simulink model "ZT_VehCtrl_18B"  (R2018b)
settings: Solver=FixedStepAuto  StartTime=0.0  StopTime=inf  FixedStep=0.005  RelTol=1e-3
InitFcn:
  | mbd_mpc_consistency_checks(bdroot(gcs));
undefined symbols (not defined in the file or in its folder): ANG_DEAD, BMS_NormalPwr, BrkPrsByBrkPct_TB_X, BrkPrsByBrkPct_TB_Y, DELAY_DISCHARGE, DELAY_RCUOFF, DRV_BACKWARD, DRV_BRAKE, DRV_FORWARD, DRV_NEUTRAL, DRV_PARK, DRV_UNPARK, DRV_ZEROTURN, EPB_LOCK, EPB_UNLOCK, ExtraLoadPwr, FanOff, fifo_0_vect, fifo_1_vect, HiFanReq, HV_finished, HV_No_Active, HV_POWER_OFF, HV_POWER_ON, HVDown, HVON, KaTLS_v_DrgUp_X_VehSpd, KeFTM_s_Way1OffDlyTime, KeFTM_TK_Way1CoolLv2OffBatTemp, KeFTM_TK_Way1CoolLv2OffMtrTemp, KeFTM_TK_Way1CoolLv2OnBatTemp, KeFTM_TK_Way1CoolLv2OnMtrTemp, KeFTM_TK_Way1CoolLv3OffBatTemp, KeFTM_TK_Way1CoolLv3OffMtrTemp, KeFTM_TK_Way1CoolLv3OnBatTemp, KeFTM_TK_Way1CoolLv3OnMtrTemp, KeFTM_TK_Way1CoolLv4OffBatTemp, KeFTM_TK_Way1CoolLv4OffMtrTemp, KeFTM_TK_Way1CoolLv4OnBatTemp, KeFTM_TK_Way1CoolLv4OnMtrTemp, Kp1, Kp2, LowFanReq, LQFP, MtrPwrFactor_RCU, MtrPwrHighToMidThd, MtrPwrLowToMidThd, MtrPwrMidToHighThd, MtrPwrMidToLowThd, MtrTrqMax, PCT_DEAD, Precharge, PTO_1000, PTO_540, pts1_fifo_0_vect, pts1_fifo_1_vect, pts2_fifo_0_vect, pts2_fifo_1_vect, pts3_fifo_0_vect, pts3_fifo_1_vect ... (+24)
libraries: mbd_mpc574x_ec_toolbox x173, canmsglib x72, simulink x57
(part 10 of 12)

== system ZT_VehCtrl_18B/SigIn/CAN1/TWV /UNPACK ==
  ID : Inport
  data : Inport  Port=2
  length : Inport  Port=3
  timestamp : Inport  Port=4
  Action Port : ActionPort
  Bus Creator : BusCreator  Inputs=7  OutDataTypeStr=Bus: CAN_MESSAGE_BUS  NonVirtualBus=on
  Bus Creator1 : BusCreator  Inputs=3
  CAN Unpack6 : canmsglib/CAN Unpack  CANdbFile=D:\VCU\VCU_SL_ZhengZhou\ZT2\模型与接口\CAN_DBC\动力CANB_GBK.dbc  MsgList=TWV  MsgName=TWV  MsgIDType=Extended (29-bit identifier)  MsgIdentifier=419374139  MsgLength=8  SignalInfo=TWV1_P_MotorOpenCircuitFlt$6$1$1$2$1$0$1$0$0$1$#TWV1_P_MotorSta$7$1$1$2$1$0$1$0$0$1$#TWV1_P_OverCurrent$2$1$1$2$1$0$1$0$0$1$#TWV1_P_OverTempFlt$3$1$1$2$1$0$1$0$0$1$#TWV1_P_OverVoltageFlt$1$1$1$2$1$0$1$0$0$1$#TWV1_P_RESP_ERROR$0$1$1$2$1$0$1$0$0$1$#TWV1_P_RealSta$8$8$1$2$1$0$4.000000e-01$0$0$100$#TWV1_P_StallFlt$5$1$1$2$1$0$1$0$0$1$#TWV1_P_UnderVoltageFlt$4$1$1$2$1$0$1$0$0$1$#  NSignals=9  IDPort=off  TimestampPort=off  ErrorPort=off  RemotePort=off  LengthPort=off  StatusPort=off  StartBits=str2num('[int32(6);int32(7);int32(2);int32(3);int32(1);int32(0);int32(8);int32(5);int32(4)]')  SignalSizes=str2num('[int32(1);int32(1);int32(1);int32(1);int32(1);int32(1);int32(8);int32(1);int32(1)]')  ByteOrders=str2num('[int32(1);int32(1);int32(1);int32(1);int32(1);int32(1);int32(1);int32(1);int32(1)]')  DataTypes=str2num('[int32(2);int32(2);int32(2);int32(2);int32(2);int32(2);int32(2);int32(2);int32(2)]')  MultiplexTypes=str2num('[int32(1);int32(1);int32(1);int32(1);int32(1);int32(1);int32(1);int32(1);int32(1)]')  MultiplexValues=str2num('[double(0);double(0);double(0);double(0);double(0);double(0);double(0);double(0);double(0)]')  Factors=str2num('[double(1);double(1);double(1);double(1);double(1);double(1);double(4.000000e-01);double(1);double(1)]')  Offsets=str2num('[double(0);double(0);double(0);double(0);double(0);double(0);double(0);double(0);double(0)]')  Minimums=str2num('[double(0);double(0);double(0);double(0);double(0);double(0);double(0);double(0);double(0)]')  Maximums=str2num('[double(1);double(1);double(1);double(1);double(1);double(1);double(100);double(1);double(1)]')  ApplyMinMax=off
      settings: SourceProductName=Simulink Real-Time  SourceProductBaseCode=XP  DataFormat=CANdb specified signals
  Constant1 : Constant  OutDataTypeStr=uint8
  Constant4 : Constant  Value=0  OutDataTypeStr=uint8
  Constant5 : Constant  Value=0  OutDataTypeStr=uint8
  Data Type Conversion{,14..15,17} (4 alike) : DataTypeConversion  OutDataTypeStr=uint8
  Data Type Conversion18 : DataTypeConversion  OutDataTypeStr=uint32
  Data Type Conversion19 : DataTypeConversion  OutDataTypeStr=double
  Message : Outport
  wires:
  Constant4/1 -> Data Type Conversion15/1
  length/1 -> Data Type Conversion14/1
  data/1 -> Bus Creator/7  "Data"
  Data Type Conversion18/1 -> Bus Creator/5  "ID"
  Constant1/1 -> Data Type Conversion/1
  Constant5/1 -> Data Type Conversion17/1
  ID/1 -> Data Type Conversion18/1
  Data Type Conversion19/1 -> Bus Creator/6  "Timestamp"
  timestamp/1 -> Data Type Conversion19/1
  Data Type Conversion17/1 -> Bus Creator/4  "Error"
  Bus Creator/1 -> CAN Unpack6/1  "CAN_Msg_In"
  Data Type Conversion/1 -> Bus Creator/1  "Extended"
  Data Type Conversion14/1 -> Bus Creator/2  "Length"
  Data Type Conversion15/1 -> Bus Creator/3  "Remote"
  Bus Creator1/1 -> Message/1

== system ZT_VehCtrl_18B/SigIn/PWM/PWM_PTS1/Subsystem ==
  In1 : Inport
  Add2 : Sum  AccumDataTypeStr=single
  Constant : Constant  OutDataTypeStr=uint8
  Constant1 : Constant  Value=0  OutDataTypeStr=single
  Data Store Read3 : DataStoreRead  DataStoreName=pts1_pwm_cnt
  Data Store Write : DataStoreWrite  DataStoreName=pts1_pwm_cnt
  Saturation : Saturate  UpperLimit=100  LowerLimit=0
  Switch : Switch  Criteria=u2 > Threshold  Threshold=100
  Out1 : Outport  VectorParamsAs1DForOutWhenUnconnected=on
  wires:
  Saturation/1 -> Data Store Write/1
  Add2/1 -> Switch/2, Saturation/1
  Data Store Read3/1 -> Add2/2
  Constant1/1 -> Switch/1
  Switch/1 -> Out1/1
  Constant/1 -> Add2/1
  In1/1 -> Switch/3

== system ZT_VehCtrl_18B/SigIn/PWM/PWM_PTS1/Subsystem_capture ==
  In1 : Inport
  function : TriggerPort  TriggerType=function-call  VariantControl=Variant
  Constant : Constant  Value=0  OutDataTypeStr=uint8
  Counter Limited : simulink/Sources/Counter Limited  uplimit=7  tsamp=-1
  Data Store Write : DataStoreWrite  DataStoreName=pts1_pwm_cnt
  Data Store Write3 : DataStoreWrite  DataStoreName=pwm3_cnt
  Terminator : Terminator
  eTimer_Arm_Capture : mbd_mpc574x_ec_toolbox/Motor Control Blocks/eTIMER Blocks/eTimer_Arm_Capture  etimerModule=1  etimerChannel=2  etimerArmAction=Stop
  eTimer_Capture : mbd_mpc574x_ec_toolbox/Motor Control Blocks/eTIMER Blocks/eTimer_Capture  etimerModule=1  etimerChannel=2
      settings: SourceProductName=NXP Model-Based Design Toolbox for MPC57xx MCUs
  Out1 : Outport  OutDataTypeStr=uint16
  Out2 : Outport  Port=2  OutDataTypeStr=uint16
  Out3 : Outport  Port=3  OutDataTypeStr=uint16
  Out4 : Outport  Port=4  OutDataTypeStr=uint16
  wires:
  eTimer_Capture/1 -> Out1/1
  eTimer_Capture/4 -> Out4/1
  eTimer_Capture/3 -> Out3/1
  eTimer_Capture/2 -> Out2/1
  In1/1 -> Terminator/1
  Constant/1 -> Data Store Write/1
  Counter Limited/1 -> Data Store Write3/1

== system ZT_VehCtrl_18B/SigIn/PWM/PWM_PTS2/Subsystem ==
  In1 : Inport
  Add2 : Sum  AccumDataTypeStr=single
  Constant : Constant  OutDataTypeStr=uint8
  Constant1 : Constant  Value=0  OutDataTypeStr=single
  Data Store Read3 : DataStoreRead  DataStoreName=pts2_pwm_cnt
  Data Store Write : DataStoreWrite  DataStoreName=pts2_pwm_cnt
  Saturation : Saturate  UpperLimit=100  LowerLimit=0
  Switch : Switch  Criteria=u2 > Threshold  Threshold=100
  Out1 : Outport  VectorParamsAs1DForOutWhenUnconnected=on
  wires:
  In1/1 -> Switch/3
  Constant/1 -> Add2/1
  Switch/1 -> Out1/1
  Constant1/1 -> Switch/1
  Data Store Read3/1 -> Add2/2
  Add2/1 -> Saturation/1, Switch/2
  Saturation/1 -> Data Store Write/1

== system ZT_VehCtrl_18B/SigIn/PWM/PWM_PTS2/Subsystem_capture ==
  In1 : Inport
  function : TriggerPort  TriggerType=function-call  VariantControl=Variant
  Constant : Constant  Value=0  OutDataTypeStr=uint8
  Counter Limited : simulink/Sources/Counter Limited  uplimit=255  tsamp=-1
  Data Store Write : DataStoreWrite  DataStoreName=pts2_pwm_cnt
  Data Store Write2 : DataStoreWrite  DataStoreName=pwm2_cnt
  Terminator : Terminator
  eTimer_Arm_Capture : mbd_mpc574x_ec_toolbox/Motor Control Blocks/eTIMER Blocks/eTimer_Arm_Capture  etimerModule=1  etimerChannel=3  etimerArmAction=Stop
  eTimer_Capture : mbd_mpc574x_ec_toolbox/Motor Control Blocks/eTIMER Blocks/eTimer_Capture  etimerModule=1  etimerChannel=3
      settings: SourceProductName=NXP Model-Based Design Toolbox for MPC57xx MCUs
  Out1 : Outport  OutDataTypeStr=uint16
  Out2 : Outport  Port=2  OutDataTypeStr=uint16
  Out3 : Outport  Port=3  OutDataTypeStr=uint16
  Out4 : Outport  Port=4  OutDataTypeStr=uint16
  wires:
  Constant/1 -> Data Store Write/1
  In1/1 -> Terminator/1
  eTimer_Capture/2 -> Out2/1
  eTimer_Capture/3 -> Out3/1
  eTimer_Capture/4 -> Out4/1
  eTimer_Capture/1 -> Out1/1
  Counter Limited/1 -> Data Store Write2/1

== system ZT_VehCtrl_18B/SigIn/PWM/PWM_PTS3/Subsystem ==
  In1 : Inport
  Add2 : Sum  AccumDataTypeStr=single
  Constant : Constant  OutDataTypeStr=uint8
  Constant1 : Constant  Value=0  OutDataTypeStr=single
  Data Store Read3 : DataStoreRead  DataStoreName=pts3_pwm_cnt
  Data Store Write : DataStoreWrite  DataStoreName=pts3_pwm_cnt
  Saturation : Saturate  UpperLimit=100  LowerLimit=0
  Switch : Switch  Criteria=u2 > Threshold  Threshold=100
  Out1 : Outport  VectorParamsAs1DForOutWhenUnconnected=on
  wires:
  Saturation/1 -> Data Store Write/1
  Add2/1 -> Switch/2, Saturation/1
  Data Store Read3/1 -> Add2/2
  Constant1/1 -> Switch/1
  Switch/1 -> Out1/1
  Constant/1 -> Add2/1
  In1/1 -> Switch/3

== system ZT_VehCtrl_18B/SigIn/PWM/PWM_PTS3/Subsystem_capture ==
  In1 : Inport
  function : TriggerPort  TriggerType=function-call  VariantControl=Variant
  Constant : Constant  Value=0  OutDataTypeStr=uint8
  Counter Limited : simulink/Sources/Counter Limited  uplimit=255  tsamp=-1
  Data Store Write : DataStoreWrite  DataStoreName=pts3_pwm_cnt
  Data Store Write4 : DataStoreWrite  DataStoreName=pwm4_cnt
  Terminator : Terminator
  eTimer_Arm_Capture : mbd_mpc574x_ec_toolbox/Motor Control Blocks/eTIMER Blocks/eTimer_Arm_Capture  etimerModule=1  etimerChannel=1  etimerArmAction=Stop
  eTimer_Capture : mbd_mpc574x_ec_toolbox/Motor Control Blocks/eTIMER Blocks/eTimer_Capture  etimerModule=1  etimerChannel=1
      settings: SourceProductName=NXP Model-Based Design Toolbox for MPC57xx MCUs
  Out1 : Outport  OutDataTypeStr=uint16
  Out2 : Outport  Port=2  OutDataTypeStr=uint16
  Out3 : Outport  Port=3  OutDataTypeStr=uint16
  Out4 : Outport  Port=4  OutDataTypeStr=uint16
  wires:
  eTimer_Capture/1 -> Out1/1
  eTimer_Capture/4 -> Out4/1
  eTimer_Capture/3 -> Out3/1
  eTimer_Capture/2 -> Out2/1
  In1/1 -> Terminator/1
  Constant/1 -> Data Store Write/1
  Counter Limited/1 -> Data Store Write4/1

== system ZT_VehCtrl_18B/SigIn/PWM/PWM_PTS4/Subsystem ==
  In1 : Inport
  Add2 : Sum  AccumDataTypeStr=single
  Constant : Constant  OutDataTypeStr=uint8
  Constant1 : Constant  Value=0  OutDataTypeStr=single
  Data Store Read3 : DataStoreRead  DataStoreName=pts4_pwm_cnt
  Data Store Write : DataStoreWrite  DataStoreName=pts4_pwm_cnt
  Saturation : Saturate  UpperLimit=100  LowerLimit=0
  Switch : Switch  Criteria=u2 > Threshold  Threshold=100
  Out1 : Outport  VectorParamsAs1DForOutWhenUnconnected=on
  wires:
  In1/1 -> Switch/3
  Constant/1 -> Add2/1
  Switch/1 -> Out1/1
  Constant1/1 -> Switch/1
  Data Store Read3/1 -> Add2/2
  Add2/1 -> Saturation/1, Switch/2
  Saturation/1 -> Data Store Write/1

== system ZT_VehCtrl_18B/SigIn/PWM/PWM_PTS4/Subsystem_capture ==
  In1 : Inport
  function : TriggerPort  TriggerType=function-call  VariantControl=Variant
  Constant : Constant  Value=0  OutDataTypeStr=uint8
  Counter Limited : simulink/Sources/Counter Limited  uplimit=255  tsamp=-1
  Data Store Write : DataStoreWrite  DataStoreName=pts4_pwm_cnt
  Data Store Write1 : DataStoreWrite  DataStoreName=pwm1_cnt
  Terminator : Terminator
  eTimer_Arm_Capture : mbd_mpc574x_ec_toolbox/Motor Control Blocks/eTIMER Blocks/eTimer_Arm_Capture  etimerModule=0  etimerChannel=2  etimerArmAction=Stop
  eTimer_Capture : mbd_mpc574x_ec_toolbox/Motor Control Blocks/eTIMER Blocks/eTimer_Capture  etimerModule=0  etimerChannel=2
      settings: SourceProductName=NXP Model-Based Design Toolbox for MPC57xx MCUs
  Out1 : Outport  OutDataTypeStr=uint16
  Out2 : Outport  Port=2  OutDataTypeStr=uint16
  Out3 : Outport  Port=3  OutDataTypeStr=uint16
  Out4 : Outport  Port=4  OutDataTypeStr=uint16
  wires:
  Constant/1 -> Data Store Write/1
  In1/1 -> Terminator/1
  eTimer_Capture/2 -> Out2/1
  eTimer_Capture/3 -> Out3/1
  eTimer_Capture/4 -> Out4/1
  eTimer_Capture/1 -> Out1/1
  Counter Limited/1 -> Data Store Write1/1

== system ZT_VehCtrl_18B/SigIn/PWM/Subsystem/Frequency_DutyCycle_Computation ==
  Add : Sum  Inputs=+-  AccumDataTypeStr=single
  Add1 : Sum  Inputs=+-  AccumDataTypeStr=single
  Data Store Read : DataStoreRead  DataStoreName=fifo_0_vect  DataStoreElements=fifo_0_vect(2)#fifo_0_vect(1)
  Data Store Read1 : DataStoreRead  DataStoreName=fifo_1_vect  DataStoreElements=fifo_1_vect(1)
  Data Store Read2 : DataStoreRead  DataStoreName=fifo_0_vect  DataStoreElements=fifo_0_vect(1)
  Divide : Product  Inputs=*/  OutDataTypeStr=single
  Divide1 : Product  Inputs=*//
  Freq_MC : Constant  Value=80000000  OutDataTypeStr=single
  Prescaler : Constant  Value=32  OutDataTypeStr=single
  Out1 : Outport
  Out2 : Outport  Port=2
  wires:
  Data Store Read1/1 -> Add1/1
  Data Store Read/2 -> Add/2
  Divide1/1 -> Out2/1
  Add/1 -> Divide/2, Divide1/3
  Add1/1 -> Divide/1
  Divide/1 -> Out1/1
  Data Store Read/1 -> Add/1
  Freq_MC/1 -> Divide1/1
  Prescaler/1 -> Divide1/2
  Data Store Read2/1 -> Add1/2

== system ZT_VehCtrl_18B/SigIn/PWM/Subsystem/eTimer Configuration and Signal Measurements ==
  Subsystem_capture : Subsystem
  eTimer_Arm_Capture : mbd_mpc574x_ec_toolbox/Motor Control Blocks/eTIMER Blocks/eTimer_Arm_Capture  etimerModule=0  etimerChannel=1  etimerArmAction=Start
  eTimer_Config : mbd_mpc574x_ec_toolbox/Motor Control Blocks/eTIMER Blocks/eTimer_Config  etimerModule=0  etimerChannel=1  etimerMode=COUNT Mode  etimerCountOnce=Count repeatedly  etimerCountLength=Continue counting to roll over  etimerCountDirection=Count up  etimerCountStart=on  etimerCaptureArm=on  etimerShowAdv=on  etimerPrimarySource=IP Bus clock divide by 32 prescaler  etimerPrimaryPolarity=True polarity  etimerSecondarySource=Counter 0 input pin  etimerSecondaryPolarity=True polarity  etimerSampleCount=Require 3 consecutive samples to be of equal value  etimerSamplePeriod=0  etimerOutEnable=The external pin is configured as an input  etimerOutPolarity=True polarity  etimerOutMode=Toggle OFLAG output using alternating compare registers  etimerCompMode="COMP1 and COMP2  are used when the counter is counting up"  etimerCompLoad1=COMP1 is never preload  etimerCompLoad2=COMP2 is never preload  etimerCapt1=Capture rising edges  etimerCapt2=Capture falling edges  etimerOneShot=Free running mode is selected  etimerMasterMode=Disable broadcast of this channel output  etimerCoForce=Other channels cannot force this channel output  etimerCoChanInit=Other channels cannot force re-initialization of this channel  etimerRedundant=off  etimerCOMP1init=0  etimerCOMP2init=0  etimerCNTRinit=0  etimerCh0=PTA0: [eTimer0_ETC0 | eTimer_0 Input Data Channel 0]  etimerCh1=None  etimerCh2=None  etimerCh3=None  etimerCh4=None  etimerCh5=None  etimerIsrTCFIE=off  etimerIsrTCF1IE=off  etimerIsrTCF2IE=off  etimerIsrTOFIE=off  etimerIsrIELFIE=off  etimerIsrIEHFIE=off  etimerIsrICF1IE=off  etimerIsrICF2IE=on  etimerIsrRCF=off  etimerIsrWDF=off
  eTimer_ISR : mbd_mpc574x_ec_toolbox/Motor Control Blocks/eTIMER Blocks/eTimer_ISR_Handler  etimerModule=0  etimerInterrupt=Channel Interrupt  etimerChannel=1  etimerIsrPriority=14
  Out1 : Outport
  Out2 : Outport  Port=2
  Out3 : Outport  Port=3
  Out4 : Outport  Port=4
  wires:
  eTimer_ISR/1 -> Subsystem_capture/Trigger
  eTimer_ISR/2 -> Subsystem_capture/1(In1)
  Subsystem_capture/1(Out1) -> Out1/1
  Subsystem_capture/2(Out2) -> Out2/1
  Subsystem_capture/3(Out3) -> Out3/1
  Subsystem_capture/4(Out4) -> Out4/1

== system ZT_VehCtrl_18B/SigOut/GPIO /ETC/Subsystem ==
  COMPLD1 : Inport
  COMPLD2 : Inport  Port=2
  Constant4 : Constant  Value=0  OutDataTypeStr=Inherit: Inherit via back propagation
  Data Type Conversion : DataTypeConversion
  Data Type Conversion1 : DataTypeConversion
  Data Type Conversion2 : DataTypeConversion
  eTimer_Preload2 : mbd_mpc574x_ec_toolbox/Motor Control Blocks/eTIMER Blocks/eTimer_Preload  etimerModule=0  etimerChannel=3
      settings: SourceProductName=NXP Model-Based Design Toolbox for MPC57xx MCUs
  eTimer_Start_Stop_Timer1 : mbd_mpc574x_ec_toolbox/Motor Control Blocks/eTIMER Blocks/eTimer_Start_Stop_Timer  etimerModule=0  etimerChannel=3  etimerAction=Start
      settings: SourceProductName=NXP Model-Based Design Toolbox for MPC57xx MCUs
  wires:
  Constant4/1 -> Data Type Conversion/1
  COMPLD2/1 -> Data Type Conversion2/1
  COMPLD1/1 -> Data Type Conversion1/1
  Data Type Conversion/1 -> eTimer_Preload2/1
  Data Type Conversion1/1 -> eTimer_Preload2/2
  Data Type Conversion2/1 -> eTimer_Preload2/3

== system ZT_VehCtrl_18B/SigOut/GPIO /ETC/Subsystem1 ==
  COMPLD1 : Inport
  COMPLD2 : Inport  Port=2
  Constant4 : Constant  Value=0  OutDataTypeStr=Inherit: Inherit via back propagation
  Data Type Conversion : DataTypeConversion
  Data Type Conversion1 : DataTypeConversion
  Data Type Conversion2 : DataTypeConversion
  eTimer_Preload2 : mbd_mpc574x_ec_toolbox/Motor Control Blocks/eTIMER Blocks/eTimer_Preload  etimerModule=2  etimerChannel=2
      settings: SourceProductName=NXP Model-Based Design Toolbox for MPC57xx MCUs
  eTimer_Start_Stop_Timer1 : mbd_mpc574x_ec_toolbox/Motor Control Blocks/eTIMER Blocks/eTimer_Start_Stop_Timer  etimerModule=2  etimerChannel=2  etimerAction=Start
      settings: SourceProductName=NXP Model-Based Design Toolbox for MPC57xx MCUs
  wires:
  COMPLD1/1 -> Data Type Conversion1/1
  COMPLD2/1 -> Data Type Conversion2/1
  Constant4/1 -> Data Type Conversion/1
  Data Type Conversion/1 -> eTimer_Preload2/1
  Data Type Conversion1/1 -> eTimer_Preload2/2
  Data Type Conversion2/1 -> eTimer_Preload2/3

== system ZT_VehCtrl_18B/SigOut/GPIO /ETC/Subsystem2 ==
  COMPLD1 : Inport
  COMPLD2 : Inport  Port=2
  Constant4 : Constant  Value=0  OutDataTypeStr=Inherit: Inherit via back propagation
  Data Type Conversion : DataTypeConversion
  Data Type Conversion1 : DataTypeConversion
  Data Type Conversion2 : DataTypeConversion
  eTimer_Preload2 : mbd_mpc574x_ec_toolbox/Motor Control Blocks/eTIMER Blocks/eTimer_Preload  etimerModule=0  etimerChannel=5
      settings: SourceProductName=NXP Model-Based Design Toolbox for MPC57xx MCUs
  eTimer_Start_Stop_Timer1 : mbd_mpc574x_ec_toolbox/Motor Control Blocks/eTIMER Blocks/eTimer_Start_Stop_Timer  etimerModule=0  etimerChannel=5  etimerAction=Start
      settings: SourceProductName=NXP Model-Based Design Toolbox for MPC57xx MCUs
  wires:
  Constant4/1 -> Data Type Conversion/1
  COMPLD2/1 -> Data Type Conversion2/1
  COMPLD1/1 -> Data Type Conversion1/1
  Data Type Conversion/1 -> eTimer_Preload2/1
  Data Type Conversion1/1 -> eTimer_Preload2/2
  Data Type Conversion2/1 -> eTimer_Preload2/3

== system ZT_VehCtrl_18B/SigOut/GPIO /ETC/Subsystem3 ==
  COMPLD1 : Inport
  COMPLD2 : Inport  Port=2
  Constant4 : Constant  Value=0  OutDataTypeStr=Inherit: Inherit via back propagation
  Data Type Conversion : DataTypeConversion
  Data Type Conversion1 : DataTypeConversion
  Data Type Conversion2 : DataTypeConversion
  eTimer_Preload2 : mbd_mpc574x_ec_toolbox/Motor Control Blocks/eTIMER Blocks/eTimer_Preload  etimerModule=1  etimerChannel=4
      settings: SourceProductName=NXP Model-Based Design Toolbox for MPC57xx MCUs
  eTimer_Start_Stop_Timer1 : mbd_mpc574x_ec_toolbox/Motor Control Blocks/eTIMER Blocks/eTimer_Start_Stop_Timer  etimerModule=1  etimerChannel=4  etimerAction=Start
      settings: SourceProductName=NXP Model-Based Design Toolbox for MPC57xx MCUs
  wires:
  Data Type Conversion2/1 -> eTimer_Preload2/3
  Data Type Conversion1/1 -> eTimer_Preload2/2
  Data Type Conversion/1 -> eTimer_Preload2/1
  COMPLD1/1 -> Data Type Conversion1/1
  COMPLD2/1 -> Data Type Conversion2/1
  Constant4/1 -> Data Type Conversion/1

== system ZT_VehCtrl_18B/SigOut/GPIO /ETC/Subsystem4 ==
  COMPLD1 : Inport
  COMPLD2 : Inport  Port=2
  Constant4 : Constant  Value=0  OutDataTypeStr=Inherit: Inherit via back propagation
  Data Type Conversion : DataTypeConversion
  Data Type Conversion1 : DataTypeConversion
  Data Type Conversion2 : DataTypeConversion
  eTimer_Preload2 : mbd_mpc574x_ec_toolbox/Motor Control Blocks/eTIMER Blocks/eTimer_Preload  etimerModule=1  etimerChannel=5
      settings: SourceProductName=NXP Model-Based Design Toolbox for MPC57xx MCUs
  eTimer_Start_Stop_Timer1 : mbd_mpc574x_ec_toolbox/Motor Control Blocks/eTIMER Blocks/eTimer_Start_Stop_Timer  etimerModule=1  etimerChannel=5  etimerAction=Start
      settings: SourceProductName=NXP Model-Based Design Toolbox for MPC57xx MCUs
  wires:
  Data Type Conversion2/1 -> eTimer_Preload2/3
  Data Type Conversion1/1 -> eTimer_Preload2/2
  Data Type Conversion/1 -> eTimer_Preload2/1
  Constant4/1 -> Data Type Conversion/1
  COMPLD2/1 -> Data Type Conversion2/1
  COMPLD1/1 -> Data Type Conversion1/1

== system ZT_VehCtrl_18B/SigOut/GPIO /ETC/Subsystem5 ==
  COMPLD1 : Inport
  COMPLD2 : Inport  Port=2
  Constant4 : Constant  Value=0  OutDataTypeStr=Inherit: Inherit via back propagation
  Data Type Conversion : DataTypeConversion
  Data Type Conversion1 : DataTypeConversion
  Data Type Conversion2 : DataTypeConversion
  eTimer_Preload2 : mbd_mpc574x_ec_toolbox/Motor Control Blocks/eTIMER Blocks/eTimer_Preload  etimerModule=1  etimerChannel=0
      settings: SourceProductName=NXP Model-Based Design Toolbox for MPC57xx MCUs
  eTimer_Start_Stop_Timer1 : mbd_mpc574x_ec_toolbox/Motor Control Blocks/eTIMER Blocks/eTimer_Start_Stop_Timer  etimerModule=1  etimerChannel=0  etimerAction=Start
      settings: SourceProductName=NXP Model-Based Design Toolbox for MPC57xx MCUs
  wires:
  Data Type Conversion2/1 -> eTimer_Preload2/3
  Data Type Conversion1/1 -> eTimer_Preload2/2
  Data Type Conversion/1 -> eTimer_Preload2/1
  COMPLD1/1 -> Data Type Conversion1/1
  COMPLD2/1 -> Data Type Conversion2/1
  Constant4/1 -> Data Type Conversion/1

== system ZT_VehCtrl_18B/SigOut/GPIO /PWM_OUT/PWM Configuration and Frequency Update ==
  In1 : Inport
  In2 : Inport  Port=2
  FlexPWM_Config : mbd_mpc574x_ec_toolbox/Motor Control Blocks/FlexPWM Blocks/FlexPWM_Config  Priority=1  pwmModule=0  pwmSubmodule=3  pwmMode=Edge aligned PWM  pwmPair=Independent  pwmCompSource=PWM23  pwmCounterInit=Local sync (PWMX)  pwmClockSource=Peripheral clock  pwmUnits=Hz  pwmFrequency=10000  pwmPeriod=8000  pwmPrescaler=Divide by 1  pwmDtUnits=Nanoseconds  pwmDtNs=50  pwmDtTicks=4  pwmReloadLogic=Full Cycle  pwmReloadFrequency=Every 1 PWM opportunity  pwmTriggeringSignal=Local force signal  pwmDutyCycleOutSim=off  pwmStartAfterInit=on  pwmShowAdvOpts=off  pwmPinA=PTA2: [PWM0_A3 | FlexPWM_0 Channel A Input/Output 3]  pwmPinB=None  pwmPolarityA=off  pwmPolarityB=off  pwmAInitialVal=0.25  pwmBInitialVal=0.25  pwmAShift=0  pwmBShift=0  trgReloadISR=off  trgVal0=off  trgVal1=off  trgVal2=off  trgVal3=off  trgVal4=off  trgVal5=off  trgReloadErrorISR=off  pwmPinFault=None  PwmFaultEnISR=off  pwmFaultEnA=off  pwmFaultEnB=off
  FlexPWM_Frequency_Update : mbd_mpc574x_ec_toolbox/Motor Control Blocks/FlexPWM Blocks/FlexPWM_Frequency_Update  Priority=1  pwmModule=0  pwmSubmodule0=off  pwmSubmodule1=off  pwmSubmodule2=off  pwmSubmodule3=on  pwmUnits=Hz
  wires:
  In1/1 -> FlexPWM_Frequency_Update/1
  In2/1 -> FlexPWM_Config/1

== system ZT_VehCtrl_18B/SigOut/GPIO /PWM_OUT/PWM Configuration and Frequency Update1 ==
  PWM A : Inport
  Fre A : Inport  Port=2
  PWM B : Inport  Port=3
  Fre B : Inport  Port=4
  Constant2 : Constant  Commented=on  Value=200
  Data Type Conversion : DataTypeConversion
  Data Type Conversion1 : DataTypeConversion
  Data Type Conversion2 : DataTypeConversion  Commented=on
  FlexPWM_Config : mbd_mpc574x_ec_toolbox/Motor Control Blocks/FlexPWM Blocks/FlexPWM_Config  Priority=1  pwmModule=0  pwmSubmodule=3  pwmMode=Center aligned PWM  pwmPair=Independent  pwmCompSource=PWM23  pwmCounterInit=Local sync (PWMX)  pwmClockSource=Peripheral clock  pwmUnits=Hz  pwmFrequency=200  pwmPeriod=25000  pwmPrescaler=Divide by 16  pwmDtUnits=Nanoseconds  pwmDtNs=50  pwmDtTicks=4  pwmReloadLogic=Full Cycle  pwmReloadFrequency=Every 1 PWM opportunity  pwmTriggeringSignal=Local force signal  pwmDutyCycleOutSim=off  pwmStartAfterInit=on  pwmShowAdvOpts=off  pwmPinA=PTD3: [PWM0_A3 | FlexPWM_0 Channel A Input/Output 3]  pwmPinB=PTD4: [PWM0_B3 | FlexPWM_0 Channel B Input/Output 3]  pwmPolarityA=off  pwmPolarityB=off  pwmAInitialVal=0.5  pwmBInitialVal=0.25  pwmAShift=0  pwmBShift=0  trgReloadISR=off  trgVal0=off  trgVal1=off  trgVal2=off  trgVal3=off  trgVal4=off  trgVal5=off  trgReloadErrorISR=off  pwmPinFault=None  PwmFaultEnISR=off  pwmFaultEnA=off  pwmFaultEnB=off
  FlexPWM_Frequency_Update : mbd_mpc574x_ec_toolbox/Motor Control Blocks/FlexPWM Blocks/FlexPWM_Frequency_Update  Priority=1  Commented=on  pwmModule=0  pwmSubmodule0=off  pwmSubmodule1=off  pwmSubmodule2=off  pwmSubmodule3=on  pwmUnits=Hz
  Terminator : Terminator
  Terminator1 : Terminator
  wires:
  Fre B/1 -> Terminator/1
  PWM A/1 -> Data Type Conversion/1
  Data Type Conversion/1 -> FlexPWM_Config/1
  PWM B/1 -> Data Type Conversion1/1
  Data Type Conversion1/1 -> FlexPWM_Config/2
  Fre A/1 -> Terminator1/1
  Constant2/1 -> Data Type Conversion2/1
  Data Type Conversion2/1 -> FlexPWM_Frequency_Update/1

== system ZT_VehCtrl_18B/SigOut/GPIO /PWM_OUT/PWM Configuration and Frequency Update4 ==
  PWM A : Inport
  Fre : Inport  Port=2
  Add : Sum  Inputs=+-
  Constant : Constant
  Constant1 : Constant  Commented=on  Value=200
  Data Type Conversion : DataTypeConversion
  Data Type Conversion1 : DataTypeConversion  Commented=on
  FlexPWM_Config : mbd_mpc574x_ec_toolbox/Motor Control Blocks/FlexPWM Blocks/FlexPWM_Config  Priority=1  pwmModule=0  pwmSubmodule=1  pwmMode=Center aligned PWM  pwmPair=Independent  pwmCompSource=PWM23  pwmCounterInit=Local sync (PWMX)  pwmClockSource=Peripheral clock  pwmUnits=Hz  pwmFrequency=200  pwmPeriod=25000  pwmPrescaler=Divide by 16  pwmDtUnits=Nanoseconds  pwmDtNs=50  pwmDtTicks=4  pwmReloadLogic=Full Cycle  pwmReloadFrequency=Every 1 PWM opportunity  pwmTriggeringSignal=Local force signal  pwmDutyCycleOutSim=off  pwmStartAfterInit=on  pwmShowAdvOpts=off  pwmPinA=PTC7: [PWM0_A1 | FlexPWM_0 Channel A Input/Output 1]  pwmPinB=None  pwmPolarityA=off  pwmPolarityB=off  pwmAInitialVal=0.25  pwmBInitialVal=0.25  pwmAShift=0  pwmBShift=0  trgReloadISR=off  trgVal0=off  trgVal1=off  trgVal2=off  trgVal3=off  trgVal4=off  trgVal5=off  trgReloadErrorISR=off  pwmPinFault=None  PwmFaultEnISR=off  pwmFaultEnA=off  pwmFaultEnB=off
  FlexPWM_Frequency_Update : mbd_mpc574x_ec_toolbox/Motor Control Blocks/FlexPWM Blocks/FlexPWM_Frequency_Update  Priority=1  Commented=on  pwmModule=0  pwmSubmodule0=off  pwmSubmodule1=on  pwmSubmodule2=off  pwmSubmodule3=off  pwmUnits=Hz
  Terminator : Terminator
  wires:
  PWM A/1 -> Add/2
  Add/1 -> Data Type Conversion/1
  Constant/1 -> Add/1
  Data Type Conversion/1 -> FlexPWM_Config/1
  Fre/1 -> Terminator/1
  Constant1/1 -> Data Type Conversion1/1
  Data Type Conversion1/1 -> FlexPWM_Frequency_Update/1

== system ZT_VehCtrl_18B/SigOut/GPIO /SPI0: LS09_14_15_16_1_2_11_4/LS_CTRL ==
  Enable : EnablePort
  Data Type Conversion3 : DataTypeConversion
  Data Type Conversion4 : DataTypeConversion
  Demux1 : Demux  Outputs=2
  If Action Subsystem1 : Subsystem  TreatAsAtomicUnit=on
  SPI_Master_Transfer_To1 : mbd_mpc574x_ec_toolbox/Communication Blocks/SPI Blocks/SPI_Master_Transfer  Priority=2  InstanceNumber=0  xfermode=Non blocking  timeout=50  spi_upd=on  WhichPCS=5
  Terminator : Terminator
  Terminator1 : Terminator
  Vector Concatenate1 : Concatenate
  wires:
  Vector Concatenate1/1 -> SPI_Master_Transfer_To1/1
  SPI_Master_Transfer_To1/1 -> Demux1/1
  Demux1/2 -> Data Type Conversion4/1
  Data Type Conversion3/1 -> Terminator/1
  Data Type Conversion4/1 -> Terminator1/1
  Demux1/1 -> Data Type Conversion3/1
  If Action Subsystem1/1(Out1) -> Vector Concatenate1/1
  If Action Subsystem1/2(Out2) -> Vector Concatenate1/2

== system ZT_VehCtrl_18B/SigOut/GPIO /SPI0: LS09_14_15_16_1_2_11_4/LS_CTRL1 ==
  Enable : EnablePort
  Data Type Conversion3 : DataTypeConversion
  Data Type Conversion4 : DataTypeConversion
  Demux1 : Demux  Outputs=2
  If Action Subsystem1 : Subsystem  TreatAsAtomicUnit=on
  SPI_Master_Transfer_To1 : mbd_mpc574x_ec_toolbox/Communication Blocks/SPI Blocks/SPI_Master_Transfer  Priority=2  InstanceNumber=0  xfermode=Non blocking  timeout=50  spi_upd=on  WhichPCS=1
  Terminator : Terminator
  Terminator1 : Terminator
  Vector Concatenate1 : Concatenate
  wires:
  Demux1/1 -> Data Type Conversion3/1
  Data Type Conversion4/1 -> Terminator1/1
  Data Type Conversion3/1 -> Terminator/1
  Demux1/2 -> Data Type Conversion4/1
  SPI_Master_Transfer_To1/1 -> Demux1/1
  Vector Concatenate1/1 -> SPI_Master_Transfer_To1/1
  If Action Subsystem1/2(Out2) -> Vector Concatenate1/2
  If Action Subsystem1/1(Out1) -> Vector Concatenate1/1

== system ZT_VehCtrl_18B/SigOut/GPIO /SPI3: LS03_06_07_08_10_12_13_17_18_19/Subsystem ==
  Enable : EnablePort
  Data Type Conversion : DataTypeConversion  OutDataTypeStr=uint8
  Data Type Conversion1 : DataTypeConversion  OutDataTypeStr=uint8
  Demux2 : Demux  Outputs=2
  SPI_Master_Transfer_To2 : mbd_mpc574x_ec_toolbox/Communication Blocks/SPI Blocks/SPI_Master_Transfer  Priority=2  InstanceNumber=3  xfermode=Non blocking  timeout=50  spi_upd=on  WhichPCS=3
  Terminator2 : Terminator
  Terminator3 : Terminator
  Vector Concatenate2 : Concatenate
  控制 : Subsystem  TreatAsAtomicUnit=on
  wires:
  Data Type Conversion1/1 -> Terminator3/1
  控制/2(Out2) -> Vector Concatenate2/2
  Demux2/1 -> Data Type Conversion/1
  Vector Concatenate2/1 -> SPI_Master_Transfer_To2/1
  Demux2/2 -> Data Type Conversion1/1
  Data Type Conversion/1 -> Terminator2/1
  控制/1(Out1) -> Vector Concatenate2/1
  SPI_Master_Transfer_To2/1 -> Demux2/1

== system ZT_VehCtrl_18B/VehCtrl/MontionControl/DriveControl/Brake ==
  VehBrkTgt : Inport
  In2 : Inport  Port=2
  1-D Lookup Table : Lookup_n-D  NumberOfTableDimensions=1  BreakpointsForDimension1=BrkPrsByBrkPct_TB_X  Table=BrkPrsByBrkPct_TB_Y  InternalRulePriority=Speed  RndMeth=Simplest  InputSameDT=on
  Bus Selector : BusSelector  OutputSignals=NonDrive
  Constant : Constant
  Gain : Gain  Gain=0.01
  Switch : Switch  Criteria=u2 > Threshold
  BrkPrsTgt : Outport
  wires:
  VehBrkTgt/1 -> Gain/1  "VehBrkTgt"
  1-D Lookup Table/1 -> BrkPrsTgt/1
  Gain/1 -> Switch/3
  Switch/1 -> 1-D Lookup Table/1
  In2/1 -> Bus Selector/1
  Bus Selector/1 -> Switch/2  "<NonDrive>"
  Constant/1 -> Switch/1

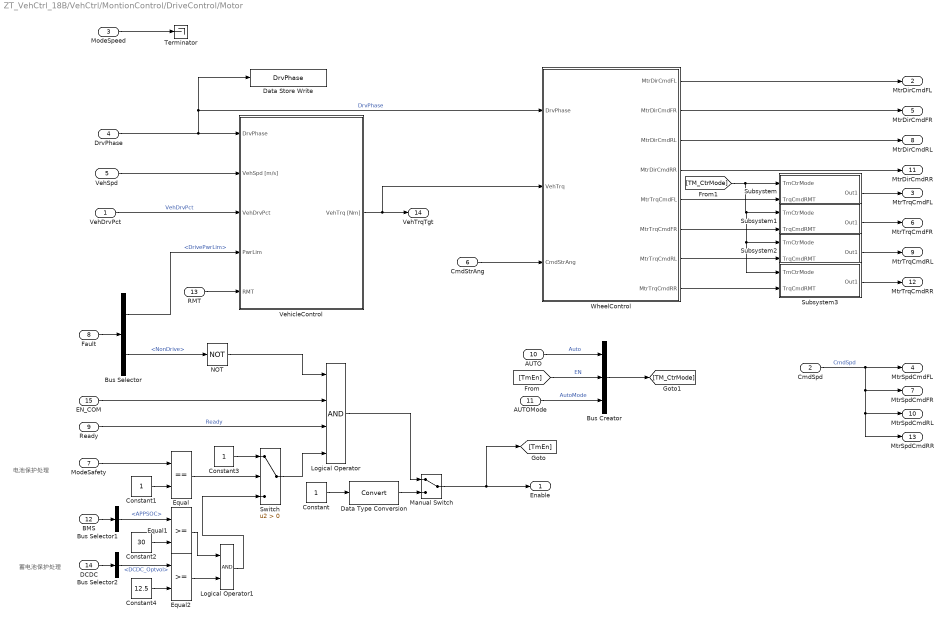
== system ZT_VehCtrl_18B/VehCtrl/MontionControl/DriveControl/Motor ==
  note: 电池保护处理
  note: 蓄电池保护处理
  VehDrvPct : Inport
  CmdSpd : Inport  Port=2
  ModeSpeed : Inport  Port=3
  DrvPhase : Inport  Port=4
  VehSpd : Inport  Port=5
  CmdStrAng : Inport  Port=6
  ModeSafety : Inport  Port=7
  Fault : Inport  Port=8
  Ready : Inport  Port=9
  AUTO : Inport  Port=10
  AUTOMode : Inport  Port=11
  BMS : Inport  Port=12
  RMT : Inport  Port=13
  DCDC : Inport  Port=14
  EN_COM : Inport  Port=15
  Bus Creator : BusCreator  Inputs=3
  Bus Selector : BusSelector  OutputSignals=DrivePwrLim,NonDrive
  Bus Selector1 : BusSelector  OutputSignals=BMS Power Infor.APPSOC
  Bus Selector2 : BusSelector  OutputSignals=DCDC_Optvol
  Constant : Constant
  Constant1 : Constant  OutDataTypeStr=boolean
  Constant2 : Constant  Value=30  OutDataTypeStr=boolean
  Constant3 : Constant  OutDataTypeStr=boolean
  Constant4 : Constant  Value=12.5  OutDataTypeStr=boolean
  Data Store Write : DataStoreWrite  DataStoreName=DrvPhase
  Data Type Conversion : DataTypeConversion
  Equal : RelationalOperator  Operator===  OutDataTypeStr=boolean  RndMeth=Simplest
  Equal1 : RelationalOperator  OutDataTypeStr=boolean  RndMeth=Simplest
  Equal2 : RelationalOperator  OutDataTypeStr=boolean  RndMeth=Simplest
  Logical Operator : Logic  Inputs=4  AllPortsSameDT=off  OutDataTypeStr=boolean
  Logical Operator1 : Logic  AllPortsSameDT=off  OutDataTypeStr=boolean
  Manual Switch : ManualSwitch
  NOT : Logic  Operator=NOT  IconShape=distinctive  AllPortsSameDT=off  OutDataTypeStr=boolean
  Subsystem : Subsystem
  Subsystem1 : Subsystem
  Subsystem2 : Subsystem
  Subsystem3 : Subsystem
  Switch : Switch  Criteria=u2 > Threshold
  Terminator : Terminator
  VehicleControl : Subsystem  TreatAsAtomicUnit=on
  WheelControl : Subsystem
  Enable : Outport
  MtrDirCmdFL : Outport  Port=2
  MtrTrqCmdFL : Outport  Port=3
  MtrSpdCmdFL : Outport  Port=4
  MtrDirCmdFR : Outport  Port=5
  MtrTrqCmdFR : Outport  Port=6
  MtrSpdCmdFR : Outport  Port=7
  MtrDirCmdRL : Outport  Port=8
  MtrTrqCmdRL : Outport  Port=9
  MtrSpdCmdRL : Outport  Port=10
  MtrDirCmdRR : Outport  Port=11
  MtrTrqCmdRR : Outport  Port=12
  MtrSpdCmdRR : Outport  Port=13
  VehTrqTgt : Outport  Port=14
  wires:
  VehSpd/1 -> VehicleControl/2(VehSpd [m/s])
  VehDrvPct/1 -> VehicleControl/3(VehDrvPct)  "VehDrvPct"
  DrvPhase/1 -> Data Store Write/1, WheelControl/1(DrvPhase), VehicleControl/1(DrvPhase)  "DrvPhase"
  CmdSpd/1 -> MtrSpdCmdRR/1, MtrSpdCmdRL/1, MtrSpdCmdFR/1, MtrSpdCmdFL/1  "CmdSpd"
  WheelControl/1(MtrDirCmdFL) -> MtrDirCmdFL/1
  WheelControl/2(MtrDirCmdFR) -> MtrDirCmdFR/1
  WheelControl/3(MtrDirCmdRL) -> MtrDirCmdRL/1
  WheelControl/4(MtrDirCmdRR) -> MtrDirCmdRR/1
  Fault/1 -> Bus Selector/1
  Bus Selector/1 -> VehicleControl/4(PwrLim)  "<DrivePwrLim>"
  Bus Selector/2 -> NOT/1  "<NonDrive>"
  NOT/1 -> Logical Operator/1
  Ready/1 -> Logical Operator/3  "Ready"
  Manual Switch/1 -> [TmEn], Enable/1
  VehicleControl/1(VehTrq [Nm]) -> WheelControl/2(VehTrq), VehTrqTgt/1
  CmdStrAng/1 -> WheelControl/3(CmdStrAng)
  WheelControl/5(MtrTrqCmdFL) -> Subsystem/2(TrqCmdRMT)
  WheelControl/6(MtrTrqCmdFR) -> Subsystem1/2(TrqCmdRMT)
  WheelControl/7(MtrTrqCmdRL) -> Subsystem2/2(TrqCmdRMT)
  WheelControl/8(MtrTrqCmdRR) -> Subsystem3/2(TrqCmdRMT)
  ModeSpeed/1 -> Terminator/1
  ModeSafety/1 -> Equal/1
  Constant1/1 -> Equal/2
  Equal/1 -> Switch/2
  Constant2/1 -> Equal1/2
  Logical Operator1/1 -> Switch/3
  Constant3/1 -> Switch/1
  Switch/1 -> Logical Operator/4
  AUTO/1 -> Bus Creator/1  "Auto"
  AUTOMode/1 -> Bus Creator/3  "AutoMode"
  BMS/1 -> Bus Selector1/1
  Bus Selector1/1 -> Equal1/1  "<APPSOC>"
  RMT/1 -> VehicleControl/5(RMT)
  Equal1/1 -> Logical Operator1/1
  Constant4/1 -> Equal2/2
  Equal2/1 -> Logical Operator1/2
  DCDC/1 -> Bus Selector2/1
  Bus Selector2/1 -> Equal2/1  "<DCDC_Optvol>"
  [TmEn] -> Bus Creator/2  "EN"
  Subsystem/1(Out1) -> MtrTrqCmdFL/1
  Bus Creator/1 -> [TM_CtrMode]
  [TM_CtrMode] -> Subsystem1/1(TmCtrMode), Subsystem3/1(TmCtrMode), Subsystem2/1(TmCtrMode), Subsystem/1(TmCtrMode)
  Subsystem1/1(Out1) -> MtrTrqCmdFR/1
  Subsystem2/1(Out1) -> MtrTrqCmdRL/1
  Subsystem3/1(Out1) -> MtrTrqCmdRR/1
  Constant/1 -> Data Type Conversion/1
  Data Type Conversion/1 -> Manual Switch/2
  Logical Operator/1 -> Manual Switch/1
  EN_COM/1 -> Logical Operator/2

== system ZT_VehCtrl_18B/VehCtrl/MontionControl/PtoControl/Subsystem ==
  ModeSpeed : Inport
  DirCmd : Inport  Port=2
  Add : Sum
  Constant : Constant  Value=16  OutDataTypeStr=uint8
  Constant1 : Constant  Value=4  OutDataTypeStr=uint8
  Constant2 : Constant  Value=32  OutDataTypeStr=uint8
  Constant3 : Constant  Value=0  OutDataTypeStr=uint8
  Switch : Switch  Criteria=u2 > Threshold
  Switch1 : Switch  Criteria=u2 > Threshold
  ModeReq : Outport
  wires:
  DirCmd/1 -> Switch/2
  Constant/1 -> Switch/1
  Constant1/1 -> Switch/3
  ModeSpeed/1 -> Switch1/2
  Constant2/1 -> Switch1/1
  Constant3/1 -> Switch1/3
  Switch1/1 -> Add/1
  Switch/1 -> Add/2
  Add/1 -> ModeReq/1

== system ZT_VehCtrl_18B/VehCtrl/MontionControl/PtoControl/Subsystem1 ==
  <RMT_PtoMode> : Inport
  Constant : Constant  Value=PTO_540
  Constant1 : Constant  Value=PTO_1000
  Constant2 : Constant  Value=540  OutDataTypeStr=single
  Constant3 : Constant  Value=1000  OutDataTypeStr=single
  Constant4 : Constant  Value=0  OutDataTypeStr=single
  Gain : Gain
  GreaterThan : RelationalOperator  Operator===  OutDataTypeStr=boolean  RndMeth=Simplest
  GreaterThan1 : RelationalOperator  Operator===  OutDataTypeStr=boolean  RndMeth=Simplest
  Switch : Switch  Criteria=u2 > Threshold
  Switch1 : Switch  Criteria=u2 > Threshold
  MtrSpdCmd : Outport
  wires:
  Switch1/1 -> Switch/3
  Constant4/1 -> Switch1/3
  Constant1/1 -> GreaterThan1/2
  GreaterThan1/1 -> Switch1/2
  Constant2/1 -> Switch/1
  Constant3/1 -> Switch1/1
  Constant/1 -> GreaterThan/2
  GreaterThan/1 -> Switch/2
  <RMT_PtoMode>/1 -> GreaterThan1/1, GreaterThan/1
  Switch/1 -> Gain/1
  Gain/1 -> MtrSpdCmd/1  "MtrSpdCmd"

== system ZT_VehCtrl_18B/VehCtrl/MontionControl/ValveControl/BrakeSys ==
  BrkPrsTgt : Inport
  BrkPrs : Inport  Port=2
  Chart : Stateflow chart  Commented=on  TreatAsAtomicUnit=on
  BrkValve : Outport
  wires:
  BrkPrs/1 -> Chart/1(BrkPrs)
  BrkPrsTgt/1 -> BrkValve/1, Chart/2(BrkPrsTgt)

== system ZT_VehCtrl_18B/VehCtrl/MontionControl/ValveControl/EpbSys ==
  EpbSt : Inport
  EpbValve : Outport
  wires:
  EpbSt/1 -> EpbValve/1

== system ZT_VehCtrl_18B/VehCtrl/MontionControl/ValveControl/PumpSys ==
  Ready : Inport
  Compare To Zero : simulink/Logic and Bit Operations/Compare To Zero  relop=>  OutDataTypeStr=boolean
  Pump : Outport
  wires:
  Compare To Zero/1 -> Pump/1
  Ready/1 -> Compare To Zero/1

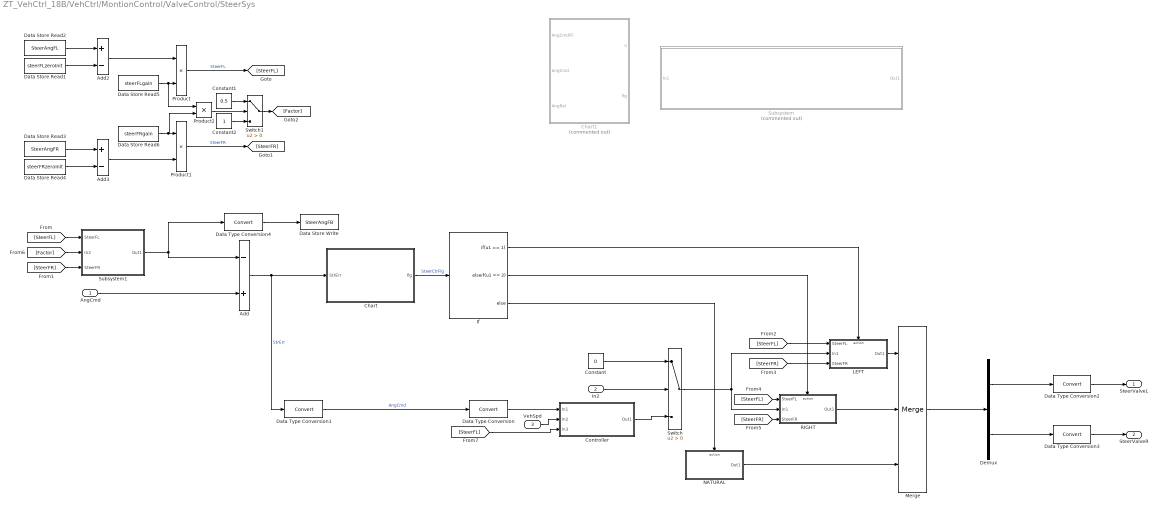
== system ZT_VehCtrl_18B/VehCtrl/MontionControl/ValveControl/SteerSys ==
  AngCmd : Inport
  In2 : Inport  Port=2
  VehSpd : Inport  Port=3
  Add : Sum  Inputs=-+
  Add2 : Sum  Inputs=+-
  Add3 : Sum  Inputs=+-
  Chart : Stateflow chart  TreatAsAtomicUnit=on
  Chart1 : Stateflow chart  Commented=on  TreatAsAtomicUnit=on
  Constant : Constant  Value=0  OutDataTypeStr=single
  Constant1 : Constant  Value=0.5  OutDataTypeStr=single
  Constant2 : Constant  OutDataTypeStr=single
  Controller : Subsystem
  Data Store Read1 : DataStoreRead  DataStoreName=steerFLzeroInit
  Data Store Read2 : DataStoreRead  DataStoreName=SteerAngFL
  Data Store Read3 : DataStoreRead  DataStoreName=SteerAngFR
  Data Store Read4 : DataStoreRead  DataStoreName=steerFRzeroInit
  Data Store Read5 : DataStoreRead  DataStoreName=steerFLgain
  Data Store Read6 : DataStoreRead  DataStoreName=steerFRgain
  Data Store Write : DataStoreWrite  DataStoreName=SteerAngFB
  Data Type Conversion{,1..4} (5 alike) : DataTypeConversion
  Demux : Demux  Outputs=2
  If : If  IfExpression=u1 == 1  ElseIfExpressions=u1 == 2
  LEFT : Subsystem  TreatAsAtomicUnit=on
  Merge : Merge  Inputs=3
  "NATURAL " : Subsystem  TreatAsAtomicUnit=on
  Product : Product
  Product1 : Product
  Product2 : Product
  RIGHT : Subsystem  TreatAsAtomicUnit=on
  Subsystem : Subsystem  Commented=on
  Subsystem1 : Subsystem
  Switch : Switch  Criteria=u2 > Threshold
  Switch1 : Switch  Criteria=u2 > Threshold
  SteerValveL : Outport
  SteerValveR : Outport  Port=2
  wires:
  If/1 -> LEFT/Action
  Switch/1 -> LEFT/2(In1), RIGHT/2(In1)
  If/2 -> RIGHT/Action
  If/3 -> "NATURAL "/Action
  RIGHT/1(Out1) -> Merge/2
  "NATURAL "/1(Out1) -> Merge/3
  LEFT/1(Out1) -> Merge/1
  Merge/1 -> Demux/1
  Data Type Conversion2/1 -> SteerValveL/1
  Data Type Conversion3/1 -> SteerValveR/1
  Demux/1 -> Data Type Conversion2/1
  Demux/2 -> Data Type Conversion3/1
  Subsystem1/1(Out1) -> Add/1, Data Type Conversion4/1
  Data Type Conversion4/1 -> Data Store Write/1
  Add/1 -> Chart/1(StrErr), Data Type Conversion1/1  "StrErr"
  Chart/1(flg) -> If/1  "SteerCtrFlg"
  Controller/1(Out1) -> Switch/3
  In2/1 -> Switch/2
  Constant/1 -> Switch/1
  AngCmd/1 -> Add/2
  VehSpd/1 -> Controller/2(In2)
  Data Type Conversion1/1 -> Data Type Conversion/1  "AngCmd"
  Add3/1 -> Product1/2
  Data Store Read4/1 -> Add3/2
  Data Store Read5/1 -> Product2/1, Product/2
  Data Store Read2/1 -> Add2/1
  Add2/1 -> Product/1
  Product1/1 -> [SteerFR]  "SteerFR"
  Data Store Read6/1 -> Product2/2, Product1/1
  Data Store Read1/1 -> Add2/2
  Data Store Read3/1 -> Add3/1
  Product/1 -> [SteerFL]  "SteerFL"
  [SteerFL] -> Subsystem1/1(SteerFL)
  [SteerFR] -> Subsystem1/3("SteerFR ")
  [SteerFR] -> LEFT/3(SteerFR)
  [SteerFL] -> LEFT/1("SteerFL ")
  [SteerFL] -> RIGHT/1(SteerFL)
  [SteerFR] -> RIGHT/3(SteerFR)
  Product2/1 -> Switch1/2
  Constant1/1 -> Switch1/1
  Constant2/1 -> Switch1/3
  Switch1/1 -> [Factor]
  [Factor] -> Subsystem1/2(In2)
  Data Type Conversion/1 -> Controller/1(In1)
  [SteerFL] -> Controller/3(In3)

== system ZT_VehCtrl_18B/VehCtrl/MontionControl/ValveControl/SuspesionSys ==
  note: 由于没有高度或长度传感器，初期为开环控制；
      | 后续考虑是否可以增加传感器，构建闭环控制。
  SuspSt : Inport
  ModeSafety : Inport  Port=2
  Constant{,1,3..4} (4 alike) : Constant  Value=false  OutDataTypeStr=boolean
  Constant2 : Constant  Value=true  OutDataTypeStr=boolean
  Constant5 : Constant  Value=true  OutDataTypeStr=boolean
  Constant6 : Constant  Value=0
  Data Type Conversion : DataTypeConversion
  Data Type Conversion1 : DataTypeConversion
  Data Type Conversion2 : DataTypeConversion  OutDataTypeStr=uint8
  Data Type Conversion3 : DataTypeConversion  OutDataTypeStr=uint8
  Data Type Conversion4 : DataTypeConversion  OutDataTypeStr=uint8
  Demux : Demux  Outputs=2
  Multiport Switch : MultiPortSwitch  DataPortOrder=Zero-based contiguous  zeroidx=on
  Mux : Mux  Inputs=2
  Mux1 : Mux  Inputs=2
  Mux2 : Mux  Inputs=2
  Switch1 : Switch  Criteria=u2 > Threshold
  SuspUpValve : Outport
  SuspDownValve : Outport  Port=2
  wires:
  Mux/1 -> Multiport Switch/2
  Mux1/1 -> Multiport Switch/3
  Mux2/1 -> Multiport Switch/4
  Constant/1 -> Mux/1
  Constant1/1 -> Mux/2
  Constant3/1 -> Mux1/2
  Constant2/1 -> Mux1/1
  Constant4/1 -> Mux2/1
  Constant5/1 -> Mux2/2
  Switch1/1 -> Data Type Conversion4/1
  Multiport Switch/1 -> Demux/1
  Demux/2 -> Data Type Conversion1/1
  Demux/1 -> Data Type Conversion/1
  Data Type Conversion/1 -> SuspUpValve/1
  Data Type Conversion1/1 -> SuspDownValve/1
  Data Type Conversion4/1 -> Multiport Switch/1  "suspmodeCtrl"
  ModeSafety/1 -> Switch1/2
  SuspSt/1 -> Data Type Conversion2/1
  Data Type Conversion2/1 -> Switch1/1
  Data Type Conversion3/1 -> Switch1/3
  Constant6/1 -> Data Type Conversion3/1

== system ZT_VehCtrl_18B/VehCtrl/MontionControl/ValveControl/WidthSys ==
  ModeSafety : Inport
  <RMT_ModeWidth> : Inport  Port=2
  Constant{,1,3..4} (4 alike) : Constant  Value=false  OutDataTypeStr=boolean
  Constant2 : Constant  Value=true  OutDataTypeStr=boolean
  Constant5 : Constant  Value=true  OutDataTypeStr=boolean
  Constant6 : Constant  Value=0  OutDataTypeStr=boolean
  Data Type Conversion : DataTypeConversion
  Data Type Conversion1 : DataTypeConversion
  Data Type Conversion2 : DataTypeConversion  OutDataTypeStr=uint8
  Data Type Conversion3 : DataTypeConversion  OutDataTypeStr=uint8
  Data Type Conversion4 : DataTypeConversion  OutDataTypeStr=uint8
  Demux : Demux  Outputs=2
  Multiport Switch : MultiPortSwitch  DataPortOrder=Zero-based contiguous  zeroidx=on
  Mux : Mux  Inputs=2
  Mux1 : Mux  Inputs=2
  Mux2 : Mux  Inputs=2
  Switch1 : Switch  Criteria=u2 > Threshold
  WidthLengthenValve : Outport
  WidthShortenValve : Outport  Port=2
  wires:
  Multiport Switch/1 -> Demux/1
  Demux/1 -> Data Type Conversion/1
  Demux/2 -> Data Type Conversion1/1
  Constant/1 -> Mux/1
  Mux2/1 -> Multiport Switch/4
  Constant2/1 -> Mux1/1
  Constant3/1 -> Mux1/2
  Mux1/1 -> Multiport Switch/3
  Mux/1 -> Multiport Switch/2
  Constant1/1 -> Mux/2
  Constant5/1 -> Mux2/2
  Constant4/1 -> Mux2/1
  Data Type Conversion/1 -> WidthLengthenValve/1
  Data Type Conversion1/1 -> WidthShortenValve/1
  ModeSafety/1 -> Switch1/2
  <RMT_ModeWidth>/1 -> Data Type Conversion2/1
  Constant6/1 -> Data Type Conversion3/1
  Switch1/1 -> Data Type Conversion4/1
  Data Type Conversion2/1 -> Switch1/1
  Data Type Conversion3/1 -> Switch1/3
  Data Type Conversion4/1 -> Multiport Switch/1  "widthmodeCtrl"

== system ZT_VehCtrl_18B/VehCtrl/TempertureControl/ThermFR_RRvRead1/Cnt_To_s ==
  In1 : Inport
  Constant1 : Constant  Value=200  OutDataTypeStr=uint8
  Data Type Conversion2 : DataTypeConversion  OutDataTypeStr=uint32
  Product1 : Product  OutDataTypeStr=fixdt(0,16,0.1,0)  RndMeth=Zero
  Out1 : Outport
  wires:
  Data Type Conversion2/1 -> Out1/1
  In1/1 -> Product1/1
  Product1/1 -> Data Type Conversion2/1
  Constant1/1 -> Product1/2

== system ZT_VehCtrl_18B/VehCtrl/TempertureControl/ThermFR_RRvRead2/Cnt_To_s ==
  In1 : Inport
  Constant1 : Constant  Value=200  OutDataTypeStr=uint8
  Data Type Conversion2 : DataTypeConversion  OutDataTypeStr=uint32
  Product1 : Product  OutDataTypeStr=fixdt(0,16,0.1,0)  RndMeth=Zero
  Out1 : Outport
  wires:
  Constant1/1 -> Product1/2
  Product1/1 -> Data Type Conversion2/1
  In1/1 -> Product1/1
  Data Type Conversion2/1 -> Out1/1

== system ZT_VehCtrl_18B/VehCtrl/TempertureControl/ThermLvRead3/Cnt_To_s ==
  In1 : Inport
  Constant1 : Constant  Value=200  OutDataTypeStr=uint8
  Data Type Conversion2 : DataTypeConversion  OutDataTypeStr=uint32
  Product1 : Product  OutDataTypeStr=fixdt(0,16,0.1,0)  RndMeth=Zero
  Out1 : Outport
  wires:
  Constant1/1 -> Product1/2
  Product1/1 -> Data Type Conversion2/1
  In1/1 -> Product1/1
  Data Type Conversion2/1 -> Out1/1

== system ZT_VehCtrl_18B/SigIn/PWM/Subsystem/eTimer Configuration and Signal Measurements/Subsystem_capture ==
  In1 : Inport
  function : TriggerPort  TriggerType=function-call  VariantControl=Variant
  Terminator : Terminator
  eTimer_Arm_Capture : mbd_mpc574x_ec_toolbox/Motor Control Blocks/eTIMER Blocks/eTimer_Arm_Capture  etimerModule=0  etimerChannel=1  etimerArmAction=Stop
  eTimer_Capture : mbd_mpc574x_ec_toolbox/Motor Control Blocks/eTIMER Blocks/eTimer_Capture  etimerModule=0  etimerChannel=1
  Out1 : Outport  OutDataTypeStr=uint16
  Out2 : Outport  Port=2  OutDataTypeStr=uint16
  Out3 : Outport  Port=3  OutDataTypeStr=uint16
  Out4 : Outport  Port=4  OutDataTypeStr=uint16
  wires:
  eTimer_Capture/1 -> Out1/1
  eTimer_Capture/4 -> Out4/1
  eTimer_Capture/3 -> Out3/1
  eTimer_Capture/2 -> Out2/1
  In1/1 -> Terminator/1

== system ZT_VehCtrl_18B/SigOut/GPIO /SPI0: LS09_14_15_16_1_2_11_4/LS_CTRL/If Action Subsystem1 ==
  Add : Sum  Inputs=++++
  Constant1 : Constant  Value=128  OutDataTypeStr=uint8
  Constant2 : Constant  Value=64  OutDataTypeStr=uint8
  Constant3 : Constant  Value=32  OutDataTypeStr=uint8
  Constant4 : Constant  Value=16  OutDataTypeStr=uint8
  Constant5 : Constant  Value=8  OutDataTypeStr=uint8
  Constant6 : Constant  Value=4  OutDataTypeStr=uint8
  Constant7 : Constant  Value=2  OutDataTypeStr=uint8
  Constant8 : Constant  OutDataTypeStr=uint8
  Constant9 : Constant  Value=128  OutDataTypeStr=uint8
  Data Store Read : DataStoreRead  DataStoreName=LS004
  Data Store Read4 : DataStoreRead  DataStoreName=LS011
  Data Store Read5 : DataStoreRead  DataStoreName=LS001
  Data Store Read6 : DataStoreRead  DataStoreName=LS002
  Data Type Conversion : DataTypeConversion
  Data Type Conversion1 : DataTypeConversion
  Switch{,1..3} (4 alike) : Switch  Criteria=u2 > Threshold
  Out1 : Outport
  Out2 : Outport  Port=2
  wires:
  Constant2/1 -> Switch/3
  Constant1/1 -> Switch/1
  Add/1 -> Data Type Conversion1/1
  Data Store Read6/1 -> Switch/2
  Constant7/1 -> Switch3/1
  Switch1/1 -> Add/2
  Constant5/1 -> Switch2/1
  Switch/1 -> Add/1
  Constant4/1 -> Switch1/3
  Data Store Read/1 -> Switch3/2
  Switch2/1 -> Add/3
  Data Store Read4/1 -> Switch2/2
  Switch3/1 -> Add/4
  Constant3/1 -> Switch1/1
  Data Store Read5/1 -> Switch1/2
  Constant8/1 -> Switch3/3
  Constant9/1 -> Data Type Conversion/1
  Constant6/1 -> Switch2/3
  Data Type Conversion/1 -> Out1/1
  Data Type Conversion1/1 -> Out2/1

== system ZT_VehCtrl_18B/SigOut/GPIO /SPI0: LS09_14_15_16_1_2_11_4/LS_CTRL1/If Action Subsystem1 ==
  Add : Sum  Inputs=++++
  Constant1 : Constant  Value=128  OutDataTypeStr=uint8
  Constant2 : Constant  Value=64  OutDataTypeStr=uint8
  Constant3 : Constant  Value=32  OutDataTypeStr=uint8
  Constant4 : Constant  Value=16  OutDataTypeStr=uint8
  Constant5 : Constant  Value=8  OutDataTypeStr=uint8
  Constant6 : Constant  Value=4  OutDataTypeStr=uint8
  Constant7 : Constant  Value=2  OutDataTypeStr=uint8
  Constant8 : Constant  OutDataTypeStr=uint8
  Constant9 : Constant  Value=128  OutDataTypeStr=uint8
  Data Store Read : DataStoreRead  DataStoreName=LS014
  Data Store Read4 : DataStoreRead  DataStoreName=LS015
  Data Store Read5 : DataStoreRead  DataStoreName=LS009
  Data Store Read6 : DataStoreRead  DataStoreName=LS016
  Data Type Conversion : DataTypeConversion
  Data Type Conversion1 : DataTypeConversion
  Switch{,1..3} (4 alike) : Switch  Criteria=u2 > Threshold
  Out1 : Outport
  Out2 : Outport  Port=2
  wires:
  Data Type Conversion1/1 -> Out2/1
  Data Type Conversion/1 -> Out1/1
  Constant6/1 -> Switch2/3
  Constant9/1 -> Data Type Conversion/1
  Constant8/1 -> Switch3/3
  Data Store Read5/1 -> Switch1/2
  Constant3/1 -> Switch1/1
  Switch3/1 -> Add/4
  Data Store Read4/1 -> Switch2/2
  Switch2/1 -> Add/3
  Data Store Read/1 -> Switch3/2
  Constant4/1 -> Switch1/3
  Switch/1 -> Add/1
  Constant5/1 -> Switch2/1
  Switch1/1 -> Add/2
  Constant7/1 -> Switch3/1
  Data Store Read6/1 -> Switch/2
  Add/1 -> Data Type Conversion1/1
  Constant1/1 -> Switch/1
  Constant2/1 -> Switch/3
